simulink model "drone_position_estimate_continuous"  (R2020b)
settings: Solver=VariableStepAuto  StartTime=0.0  StopTime=100  RelTol=1e-3
undefined symbols (not defined in the file): at, cov_an, cov_aw, cov_gps, F, g, H, L, p0, Rm, v0, x0_observer
settings Model: Creator=lucas  LastModifiedBy=lucas

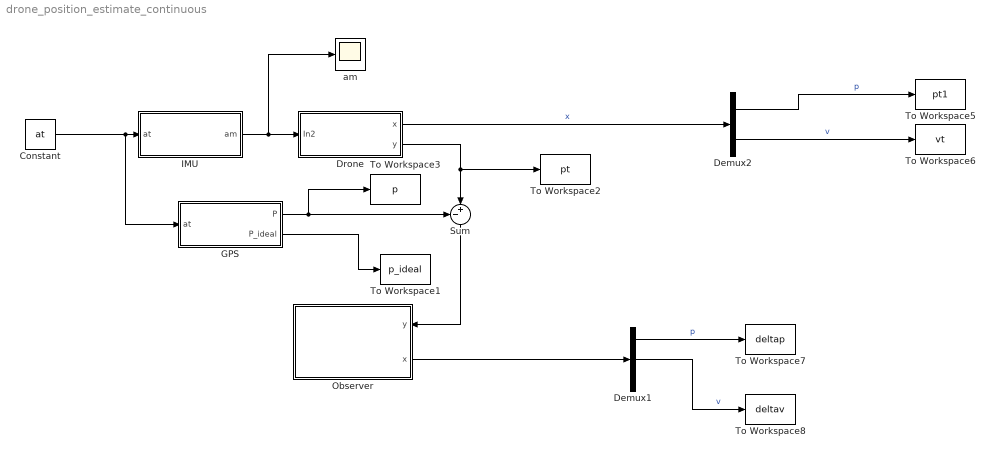
== system drone_position_estimate_continuous ==
  Constant : Constant  Value=at
  Demux1 : Demux  Outputs=3
  Demux2 : Demux  Outputs=2
  Drone : Subsystem
  GPS : Subsystem
  IMU : Subsystem
  Observer : Subsystem
      settings: PortSchema="{\"entries\":[{\"content\":{\"sides\":[{\"content\":{\"connectorIds\":[]},\"type\":\"ConnectorPlacement.EquallySpacedRectSide\",\"uuid\":\"b6dae28a-5485-44ef-84e6-2d14792229e7\"},{\"content\":{\"connectorIds\":[\"In1\",\"Out1\"],\"side\":\"RIGHT\"},\"type\":\"ConnectorPlacement.EquallySpacedRectSide\",\"uuid\":\"53a86c87-87d1-415f-9895-91b2b6ac7daf\"},{\"content\":{\"connectorIds\":[],\"side\":\"TOP\"},\"type\":\"ConnectorPlacement.EquallySpacedRectSide\",\"uuid\":\"c2916f3e-51bf-40f4-b6cd-eee6b60c38ec\"},{\"content\":{\"connectorIds\":[],\"side\":\"HIDDEN\"},\"type\":\"ConnectorPlacement.EquallySpacedRectSide\",\"uuid\":\"c85aafdf-e330-4d8d-a14a-206e12d7d836\"}]},\"type\":\"ConnectorPlacement.EquallySpacedConnector\",\"uuid\":\"08a8a426-31b9-42c2-8372-de3a4deaf2af\"}],\"packageUris\":[\"http://schema.mathworks.com/mf0/Connector/R2020b\"],\"version\":\"1.0\"}"
  Sum : Sum  Inputs=-+|
  To Workspace1 : ToWorkspace  VariableName=p_ideal  SaveFormat=Timeseries  SampleTime=-1
  To Workspace2 : ToWorkspace  VariableName=pt  SaveFormat=Timeseries  SampleTime=-1
  To Workspace3 : ToWorkspace  VariableName=p  SaveFormat=Timeseries  SampleTime=-1
  To Workspace5 : ToWorkspace  VariableName=pt1  SaveFormat=Timeseries  SampleTime=-1
  To Workspace6 : ToWorkspace  VariableName=vt  SaveFormat=Timeseries  SampleTime=-1
  To Workspace7 : ToWorkspace  VariableName=deltap  SaveFormat=Timeseries  SampleTime=-1
  To Workspace8 : ToWorkspace  VariableName=deltav  SaveFormat=Timeseries  SampleTime=-1
  am : Scope
  wires:
  IMU/1(am) -> am/1, Drone/1(In2)
  Sum/1 -> Observer/1(y)
  Drone/2(y) -> Sum/2, To Workspace2/1
  GPS/1(P) -> Sum/1, To Workspace3/1
  Demux2/1 -> To Workspace5/1  "p"
  Demux1/2 -> To Workspace8/1  "v"
  Demux2/2 -> To Workspace6/1  "v"
  Demux1/1 -> To Workspace7/1  "p"
  Observer/1(x) -> Demux1/1
  Drone/1(x) -> Demux2/1  "x"
  GPS/2(P_ideal) -> To Workspace1/1
  Constant/1 -> GPS/1(at), IMU/1(at)

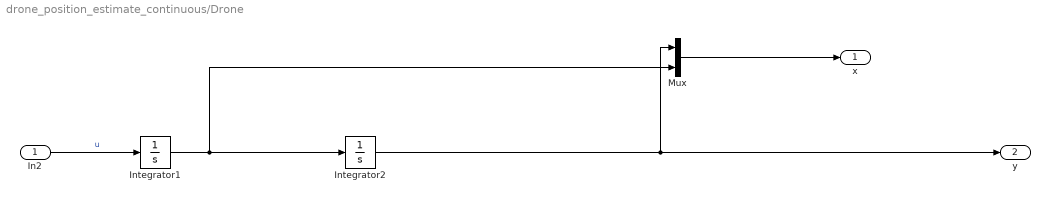
== system drone_position_estimate_continuous/Drone ==
  In2 : Inport
  Integrator1 : Integrator  InitialCondition=v0
  Integrator2 : Integrator  InitialCondition=p0
  Mux : Mux  Inputs=2
  x : Outport
  y : Outport  Port=2
  wires:
  In2/1 -> Integrator1/1  "u"
  Integrator1/1 -> Integrator2/1, Mux/2
  Integrator2/1 -> Mux/1, y/1
  Mux/1 -> x/1

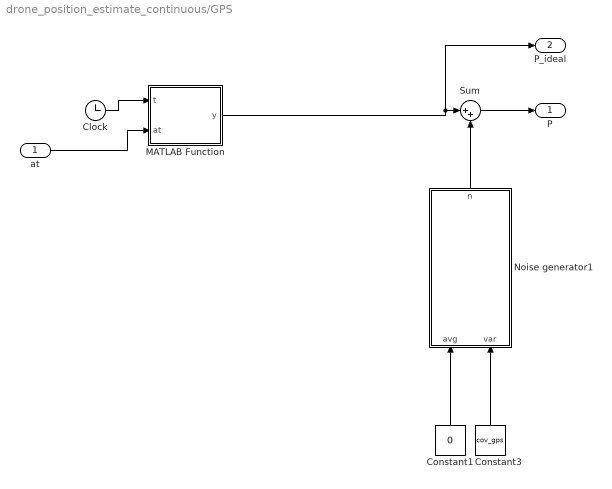
== system drone_position_estimate_continuous/GPS ==
  at : Inport
  Clock : Clock
  Constant1 : Constant  Value=0
  Constant3 : Constant  Value=cov_gps
  MATLAB Function : MATLAB Function  TreatAsAtomicUnit=on
  Noise generator1 : MATLAB Function  TreatAsAtomicUnit=on
  Sum : Sum  Inputs=|++
  P : Outport
  P_ideal : Outport  Port=2
  wires:
  Noise generator1/1(n) -> Sum/2
  Constant3/1 -> Noise generator1/2(var)
  Constant1/1 -> Noise generator1/1(avg)
  Sum/1 -> P/1
  Clock/1 -> MATLAB Function/1(t)
  MATLAB Function/1(y) -> P_ideal/1, Sum/1
  at/1 -> MATLAB Function/2(at)

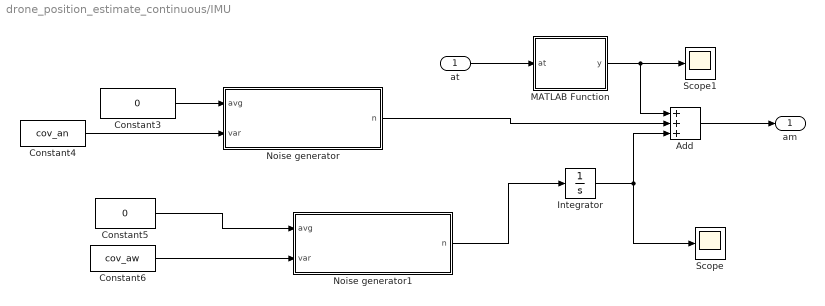
== system drone_position_estimate_continuous/IMU ==
  at : Inport
  Add : Sum  Inputs=+++
  Constant3 : Constant  Value=0  VectorParams1D=off
  Constant4 : Constant  Value=cov_an  VectorParams1D=off
  Constant5 : Constant  Value=0  VectorParams1D=off
  Constant6 : Constant  Value=cov_aw  VectorParams1D=off
  Integrator : Integrator
  MATLAB Function : MATLAB Function  TreatAsAtomicUnit=on
  Noise generator : MATLAB Function  TreatAsAtomicUnit=on
  Noise generator1 : MATLAB Function  TreatAsAtomicUnit=on
  Scope : Scope
  Scope1 : Scope
  am : Outport
  wires:
  Add/1 -> am/1
  Integrator/1 -> Scope/1, Add/3
  MATLAB Function/1(y) -> Scope1/1, Add/1
  Constant3/1 -> Noise generator/1(avg)
  Constant4/1 -> Noise generator/2(var)
  Noise generator/1(n) -> Add/2
  Constant6/1 -> Noise generator1/2(var)
  Constant5/1 -> Noise generator1/1(avg)
  Noise generator1/1(n) -> Integrator/1
  at/1 -> MATLAB Function/1(at)

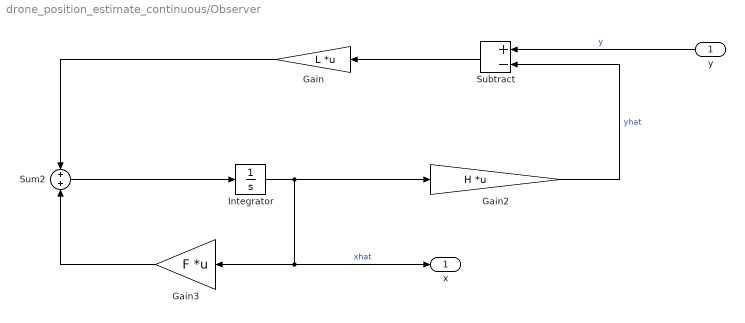
== system drone_position_estimate_continuous/Observer ==
  y : Inport
  Gain : Gain  Gain=L  Multiplication=Matrix(K*u) (u vector)
  Gain2 : Gain  Gain=H  Multiplication=Matrix(K*u) (u vector)
  Gain3 : Gain  Gain=F  Multiplication=Matrix(K*u) (u vector)
  Integrator : Integrator  InitialCondition=x0_observer
  Subtract : Sum  Inputs=+-
  Sum2 : Sum  Inputs=+|+
  x : Outport
  wires:
  Sum2/1 -> Integrator/1
  Gain3/1 -> Sum2/2
  Integrator/1 -> Gain3/1, x/1, Gain2/1  "xhat"
  y/1 -> Subtract/1  "y"
  Gain2/1 -> Subtract/2  "yhat"
  Subtract/1 -> Gain/1
  Gain/1 -> Sum2/1

== matlab function drone_position_estimate_continuous/IMU/Noise generator ==
  data: avg input; n output; var input
function n = generate_gaussian_noise(avg, var)
n = avg + var*randn(length(var), 1);

== matlab function drone_position_estimate_continuous/GPS/MATLAB Function ==
  data: t input; y output; v0 parameter; g parameter; Rm parameter; at input; p0 parameter
function y = gps_pos(t, v0, g, Rm, at, p0)
    accel = Rm*(at - g);
    y = zeros(3,1);
    for i = 1:3
        y(i) = p0(i) + (v0(i)*t) + (accel(i)*(t^2)/2);
    end

== matlab function drone_position_estimate_continuous/GPS/Noise generator1 ==
  data: avg input; n output; var input
function n = generate_gaussian_noise(avg, var)
n = avg + var*randn(length(var), 1);

== matlab function drone_position_estimate_continuous/IMU/MATLAB Function ==
  data: y output; Rm parameter; g parameter; at input
function y = fcn(Rm, g, at)
    y=Rm*(at-g);

== matlab function drone_position_estimate_continuous/IMU/Noise generator1 ==
  data: avg input; n output; var input
function n = generate_gaussian_noise(avg, var)
n = avg + var*randn(length(var), 1);
